simulink library "lib_dsphdltypes_v1"  (R2022a)
settings: Solver=ode45  StartTime=0.0  StopTime=10.0  RelTol=1e-3  EnableMultiTasking=on
libraries: simulink x7
settings Model: Creator=mbabst  LastModifiedBy=mbabst
settings SolverCC: AlgebraicLoopSolver=TrustRegion
settings DataIOCC: LimitDataPoints=on
settings OptimizationCC: LifeSpan=inf
settings DebuggingCC: UnconnectedInputMsg=warning  UnconnectedOutputMsg=warning  UnconnectedLineMsg=warning  AllowSymbolicDim=off  SFUnexpectedBacktrackingDiag=warning  SFNoUnconditionalDefaultTransitionDiag=warning  SFExecutionAtInitializationDiag=none  SFMachineParentedDataDiag=warning  ArithmeticOperatorsInVariantConditions=warning
settings SFSimCC: SimUseLocalCustomCode=off  CustomCodeUndefinedFunction=UseInterfaceOnly
settings RTWCC: RTWUseLocalCustomCode=off  DLArmComputeVersion=19.05
settings CodeAppCC: StateflowObjectComments=on
settings GRTTargetCC: TargetLangStandard=C89/C90 (ANSI)
settings ConfigComp: CovMetricSettings=dw  CovSaveCumulativeToWorkspaceVar=on  CovSaveSingleToWorkspaceVar=on  CovExternalEMLEnable=off

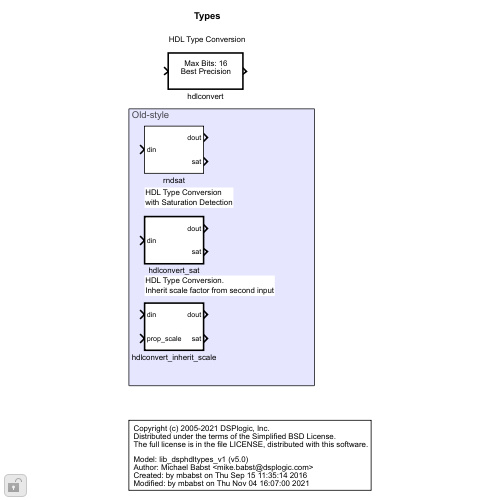
[thumbnail: Simulink's stored preview of the top-level diagram]
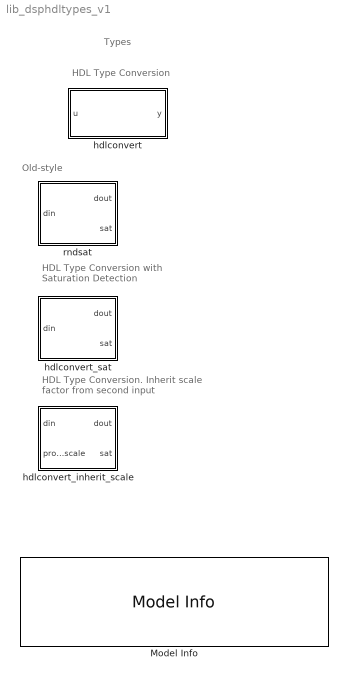
== system lib_dsphdltypes_v1 ==
  note: Types
  note: Old-style
  note: HDL Type Conversion
  note: HDL Type Conversion
      | with Saturation Detection
  note: HDL Type Conversion.
      | Inherit scale factor from second input
  Model Info : simulink/Model-Wide Utilities/Model Info  Frame=on  DisplayStringWithTags=|  HorizontalTextAlignment=Left  LeftAlignmentValue=0.02
      | Copyright (c) 2005-2021 DSPlogic, Inc.
      | Distributed under the terms of the Simplified BSD License.
      | The full license is in the file LICENSE, distributed with this software.
      | 
      | Model: %<ModelName> (v%<ModelVersion>)
      | Author: Michael Babst <mike.babst@dsplogic.com>
      | Created: by %<Creator> on %<Created>
      | Modified: by %<ModifiedBy> on %<LastModificationDate>
  hdlconvert : MATLAB Function  mask(HDL Type Conversion){signed=Inherit, maxwidth=16, extend=off, scaleopt=Best Precision, Sforce=0, roundMode=Floor, saturate=off}
      mask prompts: maxwidth "Maximum Output Width (bits)"; extend "Extend to Max Width"; scaleopt "Scale Optimization"; Sforce "Forced scale value"; roundMode "Rounding Mode"
      mask help: This block is used to convert between fixed-point types in a way that is HDL friendly. A maximum bit width can be specified with the scale factor being automatically determined based on best precision or best range requirements. Rounding and Saturation is also supported. Widths can be extended to the maximum width to help targeting fixed-precision DSP blocks. Alternately, widths can be minimized to target distributed logic.
      mask init:
      | maskstr = hdlconvert_maskstr(extend, signed, maxwidth, scaleopt, roundMode, saturate, Sforce);
  hdlconvert_inherit_scale : Subsystem  TreatAsAtomicUnit=on  mask(Hardware rounding and saturation){outSigned=on, outWidth=16, holdSaturate=on, roundMode=Nearest}
      mask prompts: outSigned "Signed"; outWidth "Output Width"; holdSaturate "Hold Saturation Event"; roundMode "Round Mode"
      mask help: Hardware rounding and saturation. Includes saturation detection.
      mask init:
      | set_param([gcb '/prop'],'SlopeBase', 'Slope1');
      settings: PermitHierarchicalResolution=None  RTWSystemCode=Inline
      mask Help:
      | Author: Mike Babst <mikebabst@gmail.com>
      | Copyright 2016 DSPlogic
      mask TypeOptions roundMode: Nearest | Floor | Convergent
      mask Callback roundMode:
      | roundMode = get_param(gcb, 'roundMode');
      | 
      | set_param([gcb '/convert'],'RndMeth', roundMode)
      mask DialogControl Control2 Prompt: Output Data Type
      mask DialogControl Container4 Prompt: Behavior
  hdlconvert_sat : Subsystem  TreatAsAtomicUnit=on  mask(Hardware rounding and saturation){outSigned=on, outWidth=16, holdSaturate=on, roundMode=Nearest, scalingSelect=Best Range, specPrecision=15}
      mask prompts: outSigned "Signed"; outWidth "Output Width"; holdSaturate "Hold Saturation Event"; roundMode "Round Mode"; scalingSelect "Scaling"; specPrecision "Output Precision"
      mask help: Hardware rounding and saturation. Includes saturation detection.
      settings: PermitHierarchicalResolution=None  RTWSystemCode=Inline
      mask Help:
      | Author: Mike Babst <mikebabst@gmail.com>
      | Copyright 2016 DSPlogic
      mask TypeOptions roundMode: Nearest | Floor | Convergent
      mask Callback roundMode:
      | roundMode = get_param(gcb, 'roundMode');
      | 
      | set_param([gcb '/convert'],'RndMeth', roundMode)
      mask TypeOptions scalingSelect: Best Range | Best Precision | Specify Precision
      mask Callback scalingSelect:
      | scalingSelect = get_param(gcb, 'scalingSelect');
      | 
      | if strcmp(scalingSelect, 'Specify Precision');
      | 
      |     set_param(gcb,'MaskVisibilities',{'on';'on';'on';'on';'on';'on'});
      | 
      |     set_param([gcb '/prop'],'SlopeBase', 'Slope1');
      | 
      | elseif strcmp(scalingSelect, 'Best Range');
      | 
      |     set_param(gcb,'MaskVisibilities',{'on';'on';'on';'on';'on';'off'});
      | 
      |     set_param([gcb '/prop'],'SlopeBase', 'PosRange2');
      | 
      | elseif strcmp(scalingSelect, 'Best Precision'),
      | 
      |     set_param(gcb,'MaskVisibilities',{'on';'on';'on';'on';'on';'off'});
      | 
      |     set_param([gcb '/prop'],'SlopeBase', 'Slope2');
      | 
      | 
      | else
      |     error('Invalid scaling mode');
      | end
      mask DialogControl Control2 Prompt: Output Data Type
      mask DialogControl Container4 Prompt: Behavior
  rndsat : Subsystem  mask(Hardware rounding and saturation){outSigned=on, outWidth=16, holdSaturate=on, roundMode=Nearest, scalingSelect=Best Range, specPrecision=15}
      mask prompts: outSigned "Signed"; outWidth "Output Width"; holdSaturate "Hold Saturation Event"; roundMode "Round Mode"; scalingSelect "Scaling"; specPrecision "Output Precision"
      mask help: Hardware rounding and saturation. Includes saturation detection.
      settings: PermitHierarchicalResolution=None  RTWSystemCode=Inline
      mask Help:
      | Author: Mike Babst <mikebabst@gmail.com>
      | Copyright 2016 DSPlogic
      mask TypeOptions roundMode: Nearest | Floor | Convergent
      mask Callback roundMode:
      | roundMode = get_param(gcb, 'roundMode');
      | 
      | set_param([gcb '/convert'],'RndMeth', roundMode)
      mask TypeOptions scalingSelect: Best Range | Best Precision | Specify Precision
      mask Callback scalingSelect:
      | scalingSelect = get_param(gcb, 'scalingSelect');
      | 
      | if strcmp(scalingSelect, 'Specify Precision');
      | 
      |     set_param(gcb,'MaskVisibilities',{'on';'on';'on';'on';'on';'on'});
      | 
      |     set_param([gcb '/prop'],'SlopeBase', 'Slope1');
      | 
      | elseif strcmp(scalingSelect, 'Best Range');
      | 
      |     set_param(gcb,'MaskVisibilities',{'on';'on';'on';'on';'on';'off'});
      | 
      |     set_param([gcb '/prop'],'SlopeBase', 'PosRange2');
      | 
      | elseif strcmp(scalingSelect, 'Best Precision'),
      | 
      |     set_param(gcb,'MaskVisibilities',{'on';'on';'on';'on';'on';'off'});
      | 
      |     set_param([gcb '/prop'],'SlopeBase', 'Slope2');
      | 
      | 
      | else
      |     error('Invalid scaling mode');
      | end
      mask DialogControl Control2 Prompt: Output Data Type
      mask DialogControl Container4 Prompt: Behavior

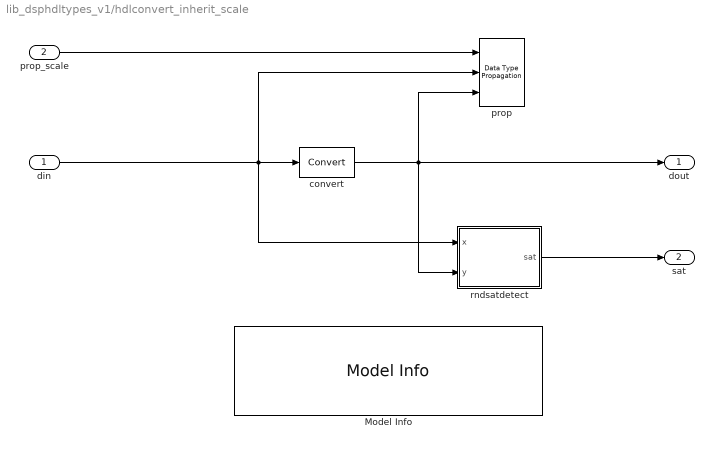
== system lib_dsphdltypes_v1/hdlconvert_inherit_scale ==
  din : Inport
  prop_scale : Inport  Port=2
  Model Info : simulink/Model-Wide Utilities/Model Info  Frame=on  DisplayStringWithTags=|  HorizontalTextAlignment=Left  LeftAlignmentValue=0.02
      | Copyright (c) 2005-2021 DSPlogic, Inc.
      | Distributed under the terms of the Simplified BSD License.
      | The full license is in the file LICENSE, distributed with this software.
      | 
      | Model: %<ModelName> (v%<ModelVersion>)
      | Author: Michael Babst <mike.babst@dsplogic.com>
      | Created: by %<Creator> on %<Created>
      | Modified: by %<ModifiedBy> on %<LastModificationDate>
  convert : DataTypeConversion  RndMeth=Nearest
  prop : simulink/Signal Attributes/Data Type Propagation  PropDataType=fixdt(1, 16)  IfRefDouble=double  IfRefSingle=single  IsSigned=IsSigned1  NumBitsBase=NumBits1  NumBitsMult=1  NumBitsAdd=0  NumBitsAllowFinal=1:128  PropScaling=2^-10  ValuesUsedBestPrec=[5 -7]  SlopeBase=Slope1  SlopeMult=1  SlopeAdd=0  BiasBase=Bias1  BiasMult=1  BiasAdd=0
      settings: SourceProductBaseCode=SL
  rndsatdetect : MATLAB Function  TreatAsAtomicUnit=on
  dout : Outport
  sat : Outport  Port=2
  wires:
  din/1 -> rndsatdetect/1(x), convert/1, prop/2
  convert/1 -> rndsatdetect/2(y), dout/1, prop/3
  rndsatdetect/1(sat) -> sat/1
  prop_scale/1 -> prop/1

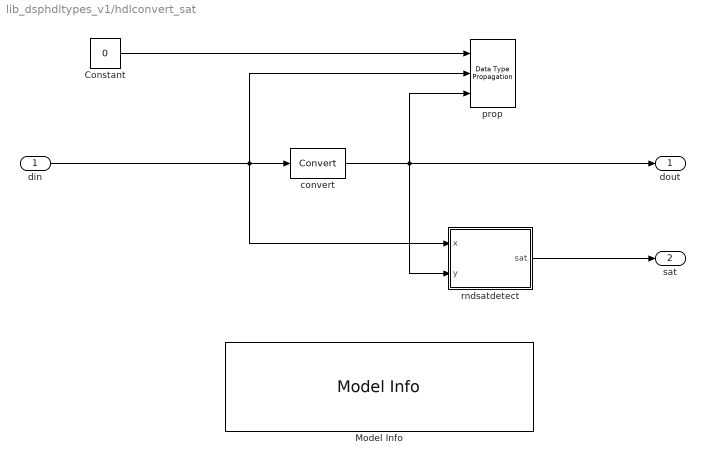
== system lib_dsphdltypes_v1/hdlconvert_sat ==
  din : Inport
  Constant : Constant  Value=0  OutDataTypeStr=fixdt(outSigned,outWidth,specPrecision)  LockScale=on
  Model Info : simulink/Model-Wide Utilities/Model Info  Frame=on  DisplayStringWithTags=|  HorizontalTextAlignment=Left  LeftAlignmentValue=0.02
      | Copyright (c) 2005-2021 DSPlogic, Inc.
      | Distributed under the terms of the Simplified BSD License.
      | The full license is in the file LICENSE, distributed with this software.
      | 
      | Model: %<ModelName> (v%<ModelVersion>)
      | Author: Michael Babst <mike.babst@dsplogic.com>
      | Created: by %<Creator> on %<Created>
      | Modified: by %<ModifiedBy> on %<LastModificationDate>
  convert : DataTypeConversion  RndMeth=Nearest
  prop : simulink/Signal Attributes/Data Type Propagation  PropDataType=fixdt(1, 16)  IfRefDouble=double  IfRefSingle=single  IsSigned=IsSigned1  NumBitsBase=NumBits1  NumBitsMult=1  NumBitsAdd=0  NumBitsAllowFinal=1:128  PropScaling=2^-10  ValuesUsedBestPrec=[5 -7]  SlopeBase=PosRange2  SlopeMult=1  SlopeAdd=0  BiasBase=Bias1  BiasMult=1  BiasAdd=0
      settings: SourceProductBaseCode=SL
  rndsatdetect : MATLAB Function  TreatAsAtomicUnit=on
  dout : Outport
  sat : Outport  Port=2
  wires:
  din/1 -> rndsatdetect/1(x), convert/1, prop/2
  convert/1 -> rndsatdetect/2(y), dout/1, prop/3
  Constant/1 -> prop/1
  rndsatdetect/1(sat) -> sat/1

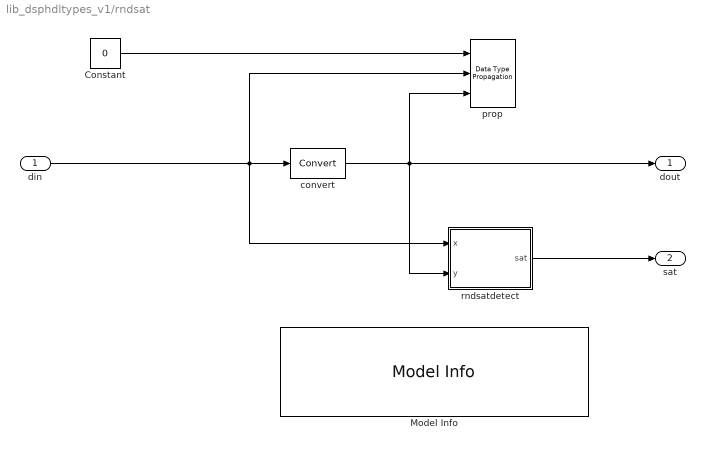
== system lib_dsphdltypes_v1/rndsat ==
  din : Inport
  Constant : Constant  Value=0  OutDataTypeStr=fixdt(outSigned,outWidth,specPrecision)  LockScale=on
  Model Info : simulink/Model-Wide Utilities/Model Info  Frame=on  DisplayStringWithTags=|  HorizontalTextAlignment=Left  LeftAlignmentValue=0.02
      | Copyright (c) 2005-2021 DSPlogic, Inc.
      | Distributed under the terms of the Simplified BSD License.
      | The full license is in the file LICENSE, distributed with this software.
      | 
      | Model: %<ModelName> (v%<ModelVersion>)
      | Author: Michael Babst <mike.babst@dsplogic.com>
      | Created: by %<Creator> on %<Created>
      | Modified: by %<ModifiedBy> on %<LastModificationDate>
  convert : DataTypeConversion  RndMeth=Nearest
  prop : simulink/Signal Attributes/Data Type Propagation  PropDataType=fixdt(1, 16)  IfRefDouble=double  IfRefSingle=single  IsSigned=IsSigned1  NumBitsBase=NumBits1  NumBitsMult=1  NumBitsAdd=0  NumBitsAllowFinal=1:128  PropScaling=2^-10  ValuesUsedBestPrec=[5 -7]  SlopeBase=PosRange2  SlopeMult=1  SlopeAdd=0  BiasBase=Bias1  BiasMult=1  BiasAdd=0
      settings: SourceProductBaseCode=SL
  rndsatdetect : MATLAB Function  TreatAsAtomicUnit=on
  dout : Outport
  sat : Outport  Port=2
  wires:
  din/1 -> rndsatdetect/1(x), convert/1, prop/2
  convert/1 -> rndsatdetect/2(y), dout/1, prop/3
  Constant/1 -> prop/1
  rndsatdetect/1(sat) -> sat/1

== matlab function lib_dsphdltypes_v1/hdlconvert_inherit_scale/rndsatdetect ==
  data: x input; y input; sat output; holdSaturate parameter
function sat = fcn(x, y, holdSaturate)
%#codegen

sat = satdetect(x,y, holdSaturate);

end

== matlab function lib_dsphdltypes_v1/hdlconvert_sat/rndsatdetect ==
  data: x input; y input; sat output; holdSaturate parameter
function sat = fcn(x, y, holdSaturate)
%#codegen

sat = satdetect(x,y, holdSaturate);

end

== matlab function lib_dsphdltypes_v1/hdlconvert ==
  data: u input; y output; extend parameter; signed parameter; maxwidth parameter; scaleopt parameter; roundMode parameter; saturate parameter; Sforce parameter
function y = hdlconvert(u, extend, signed, maxwidth, scaleopt, roundMode, saturate, Sforce) 
%#codegen
y = hdlconvert(u, extend, signed, maxwidth, scaleopt, roundMode, saturate, Sforce); 

end

== matlab function lib_dsphdltypes_v1/rndsat/rndsatdetect ==
  data: x input; y input; sat output; holdSaturate parameter
function sat = fcn(x, y, holdSaturate)
%#codegen

sat = satdetect(x,y, holdSaturate);

end
